simulink model "sampleModel1505"  (R2023a)
settings: Solver=VariableStepAuto  StartTime=0.0  StopTime=10.0  RelTol=1e-3
libraries: hdlsllib x11, simulink x2
settings Model: Creator=user1  LastModifiedBy=user1

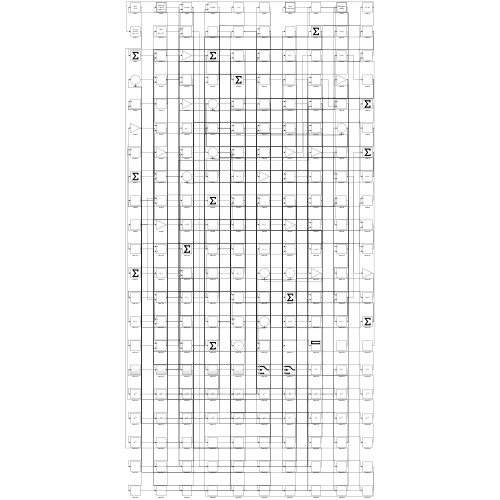
[thumbnail: Simulink's stored preview of the top-level diagram]
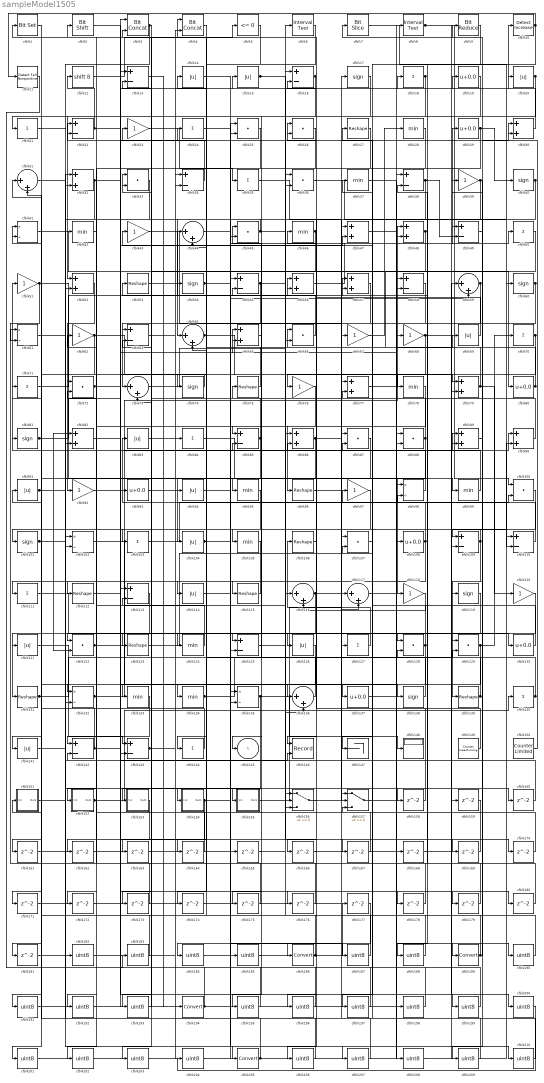
== system sampleModel1505 ==
  cfblk1 : simulink/Logic and Bit Operations/Bit Set  iBit=0
      settings: LibrarySourceBlock=|
      | hdlsllib/Logic and Bit
      | Operations/Bit Set
  cfblk10 : simulink/Logic and Bit Operations/Detect Increase  vinit=0.0  OutDataTypeStr=boolean
      settings: LibrarySourceBlock=|
      | hdlsllib/Logic and Bit
      | Operations/Detect
      | Increase
  cfblk{25..26,33,36,45,66,72,87..88,100,107,122,128..129} (14 alike) : DotProduct  OutDataTypeStr=Inherit: Inherit via internal rule
  cfblk{17,40,54,60,74,81,101,119,138} (9 alike) : Signum
  cfblk{41,61,98,102,132,135} (6 alike) : Product  Inputs=*/  RndMeth=Zero  SaturateOnIntegerOverflow=on
  cfblk{18,21,24,35,50,70..71,84,103,111,127,140,144} (13 alike) : Sum  Inputs=+
  cfblk{14..15,20,69,83,91,94,104,114,121,126,141} (12 alike) : Abs  SaturateOnIntegerOverflow=off
  cfblk{28,37,42,46,78,95,99,105,124,133..134} (11 alike) : MinMax
  cfblk{27,53,75,96,106,112,115,123,131,139} (10 alike) : Reshape
  cfblk{19,29,80,93,108,130,137} (7 alike) : Bias  Bias=0.0  SaturateOnIntegerOverflow=off
  cfblk{13,16,22,34,38,49,55,58,63,85,109..110,113,125,142..143} (16 alike) : Sum  Inputs=+-
  cfblk11 : hdlsllib/Logic and Bit Operations/Detect Fall Nonpositive  vinit=0  OutDataTypeStr=boolean
  cfblk{31,44,59,64,73,116..117,136} (8 alike) : Sum  Inputs=|++
  cfblk{23,39,43,51,62,67..68,76,92,97,118,120} (12 alike) : Gain
  cfblk12 : ArithShift  BitShiftNumber=8
  cfblk146 : Record  FileSettingsInternal="{\"entries\":[{\"content\":{\"excelSettings\":{\"content\":{},\"type\":\"Streamout.ExcelSettings\"}},\"type\":\"Streamout.FileSettingStorage\",\"uuid\":\"\"}],\"packageUris\":[\"http:\\/\\/schema.mathworks.com\\/mf0\\/streamout_blocks\\/R2020a\"],\"version\":\"1.0\"}"  Layout=[1 1]  SignalsInternal="{\"entries\":[{\"content\":{\"signals\":[{\"content\":{\"blockPath\":[],\"dimensions\":[1],\"domain\":\"\",\"lineColor\":\"#a2142f\",\"plots\":[1],\"port\":1,\"signalID\":1371,\"signalName\":\"XY Graph:1\"},\"type\":\"RecordBlkView.Signal\",\"uuid\":\"\"},{\"content\":{\"blockPath\":[],\"dimensions\":[1],\"domain\":\"\",\"lineColor\":\"#139fff\",\"plots\":[1],\"port\":2,\"signalID\":1374,\"signalName\":\"XY Graph:2\"},\"type\":\"RecordBlkView.Signal\",\"uuid\":\"\"}]},\"type\":\"RecordBlkView.InputSignals\",\"uuid\":\"\"}],\"packageUris\":[\"http:\\/\\/schema.mathworks.com\\/mf0\\/streamout_blocks\\/R2020a\"],\"version\":\"1.0\"}"  VisualizationBindings="{\"xyplotplugin\":{\"info\":[{\"series\":[{\"bindingParametersList\":[{\"parameter\":\"X-Axis\",\"signalID\":1371,\"signalName\":\"XY Graph:1\"},{\"parameter\":\"Y-Axis\",\"signalID\":1374,\"signalName\":\"XY Graph:2\"}],\"seriesID\":50908}],\"subplotID\":1}]}}"  CompatibilityTag=XY  st=-1
  cfblk147 : Terminator
  cfblk148 : Display
  cfblk149 : hdlsllib/Sources/Counter Free-Running  NumBits=16  tsamp=-1
  cfblk150 : hdlsllib/Sources/Counter Limited  uplimit=7  tsamp=-1
  cfblk151 : Subsystem
      settings: LibrarySourceBlock=|
      | hdlsllib/Ports &
      | Subsystems/Subsystem
  cfblk152 : Subsystem
      settings: LibrarySourceBlock=|
      | hdlsllib/Ports &
      | Subsystems/Subsystem
  cfblk153 : Subsystem
      settings: LibrarySourceBlock=|
      | hdlsllib/Ports &
      | Subsystems/Subsystem
  cfblk154 : Subsystem
      settings: LibrarySourceBlock=|
      | hdlsllib/Ports &
      | Subsystems/Subsystem
  cfblk155 : Subsystem
      settings: LibrarySourceBlock=|
      | hdlsllib/Ports &
      | Subsystems/Subsystem
  cfblk156 : Switch  SaturateOnIntegerOverflow=off  InputSameDT=off
  cfblk157 : Switch  SaturateOnIntegerOverflow=off  InputSameDT=off
  cfblk{158..181} (24 alike) : Delay  SampleTime=1
  cfblk{182..185,187..188,190..193,195..204,206..210} (25 alike) : DataTypeConversion  OutDataTypeStr=uint8  SaturateOnIntegerOverflow=off  RndMeth=Floor
  cfblk{186,189,194,205} (4 alike) : DataTypeConversion  SaturateOnIntegerOverflow=off  RndMeth=Floor
  cfblk2 : hdlsllib/Logic and Bit Operations/Bit Shift  mode=Shift Left Logical  N=0
  cfblk3 : hdlsllib/Logic and Bit Operations/Bit Concat  numInputs=2
  cfblk{30,32,47..48,52,56..57,65,77,79,82,86,89..90} (14 alike) : Sum
  cfblk4 : hdlsllib/Logic and Bit Operations/Bit Concat  numInputs=2
  cfblk5 : hdlsllib/Logic and Bit Operations/Compare To Zero  relop=<=  OutDataTypeStr=boolean
  cfblk6 : hdlsllib/Logic and Bit Operations/Interval Test  IntervalClosedRight=on  uplimit=0.5  IntervalClosedLeft=on  lowlimit=-0.5  OutDataTypeStr=boolean
  cfblk7 : hdlsllib/Logic and Bit Operations/Bit Slice  lidx=7  ridx=0
  cfblk8 : hdlsllib/Logic and Bit Operations/Interval Test  IntervalClosedRight=on  uplimit=0.5  IntervalClosedLeft=on  lowlimit=-0.5  OutDataTypeStr=boolean
  cfblk9 : hdlsllib/Logic and Bit Operations/Bit Reduce  mode=AND
  cfblk145 : Outport  VectorParamsAs1DForOutWhenUnconnected=off
  wires:
  cfblk52/1 -> cfblk92/1
  cfblk152/1(Out1) -> cfblk140/1, cfblk146/2, cfblk179/1
  cfblk67/1 -> cfblk28/1
  cfblk102/1 -> cfblk138/1
  cfblk103/1 -> cfblk97/1
  cfblk135/1 -> cfblk148/1, cfblk153/1(In1)
  cfblk91/1 -> cfblk99/1, cfblk122/2, cfblk82/1
  cfblk85/1 -> cfblk104/1, cfblk54/1
  cfblk140/1 -> cfblk75/1, cfblk129/2
  cfblk23/1 -> cfblk35/1
  cfblk48/1 -> cfblk65/1, cfblk128/1
  cfblk30/1 -> cfblk10/1
  cfblk19/1 -> cfblk52/1
  cfblk10/1 -> cfblk11/1, cfblk188/1
  cfblk137/1 -> cfblk50/1
  cfblk55/1 -> cfblk73/1, cfblk129/1
  cfblk90/1 -> cfblk33/1
  cfblk96/1 -> cfblk157/1
  cfblk149/1 -> cfblk53/1
  cfblk132/1 -> cfblk48/1, cfblk199/1
  cfblk70/1 -> cfblk76/1, cfblk79/1
  cfblk75/1 -> cfblk22/1
  cfblk150/1 -> cfblk7/1
  cfblk13/1 -> cfblk194/1
  cfblk38/1 -> cfblk64/1, cfblk49/2
  cfblk41/1 -> cfblk80/1
  cfblk93/1 -> cfblk18/1
  cfblk111/1 -> cfblk125/1
  cfblk53/1 -> cfblk127/1
  cfblk12/1 -> cfblk5/1
  cfblk26/1 -> cfblk144/1
  cfblk3/1 -> cfblk133/1, cfblk132/2
  cfblk110/1 -> cfblk46/1
  cfblk43/1 -> cfblk117/1
  cfblk31/1 -> cfblk205/1
  cfblk8/1 -> cfblk100/1, cfblk190/1
  cfblk127/1 -> cfblk106/1
  cfblk71/1 -> cfblk44/1
  cfblk81/1 -> cfblk65/2, cfblk160/1
  cfblk56/1 -> cfblk29/1
  cfblk73/1 -> cfblk6/1
  cfblk51/1 -> cfblk118/1, cfblk61/2
  cfblk123/1 -> cfblk17/1
  cfblk21/1 -> cfblk52/2
  cfblk64/1 -> cfblk117/2, cfblk79/2
  cfblk7/1 -> cfblk60/1
  cfblk40/1 -> cfblk63/1, cfblk156/3, cfblk195/1
  cfblk9/1 -> cfblk137/1
  cfblk46/1 -> cfblk73/2, cfblk103/1
  cfblk121/1 -> cfblk143/1
  cfblk80/1 -> cfblk4/1, cfblk66/1
  cfblk66/1 -> cfblk56/1
  cfblk130/1 -> cfblk43/1
  cfblk72/1 -> cfblk134/1, cfblk126/1
  cfblk74/1 -> cfblk72/1
  cfblk129/1 -> cfblk147/1, cfblk70/1, cfblk175/1
  cfblk35/1 -> cfblk67/1
  cfblk139/1 -> cfblk9/1, cfblk38/2
  cfblk15/1 -> cfblk169/1, cfblk170/1
  cfblk88/1 -> cfblk125/2, cfblk63/2
  cfblk45/1 -> cfblk42/1, cfblk136/2
  cfblk124/1 -> cfblk62/1
  cfblk37/1 -> cfblk189/1
  cfblk120/1 -> cfblk122/1
  cfblk4/1 -> cfblk74/1
  cfblk89/1 -> cfblk109/1
  cfblk101/1 -> cfblk201/1, cfblk207/1
  cfblk116/1 -> cfblk131/1, cfblk89/1, cfblk163/1
  cfblk112/1 -> cfblk47/2
  cfblk106/1 -> cfblk56/2
  cfblk29/1 -> cfblk95/1, cfblk40/1
  cfblk104/1 -> cfblk30/2, cfblk176/1
  cfblk24/1 -> cfblk130/1
  cfblk76/1 -> cfblk96/1
  cfblk39/1 -> cfblk108/1, cfblk136/1, cfblk119/1
  cfblk16/1 -> cfblk102/2, cfblk32/2
  cfblk94/1 -> cfblk90/1
  cfblk34/1 -> cfblk3/2
  cfblk63/1 -> cfblk57/1
  cfblk61/1 -> cfblk154/1(In1)
  cfblk6/1 -> cfblk44/2
  cfblk42/1 -> cfblk22/2
  cfblk69/1 -> cfblk26/1
  cfblk155/1(Out1) -> cfblk49/1
  cfblk22/1 -> cfblk78/1, cfblk12/1
  cfblk156/1 -> cfblk19/1
  cfblk118/1 -> cfblk116/2
  cfblk2/1 -> cfblk143/2
  cfblk115/1 -> cfblk114/1
  cfblk138/1 -> cfblk45/1
  cfblk143/1 -> cfblk34/2, cfblk20/1
  cfblk84/1 -> cfblk156/1
  cfblk99/1 -> cfblk58/1
  cfblk1/1 -> cfblk111/1
  cfblk60/1 -> cfblk88/2, cfblk124/1
  cfblk87/1 -> cfblk186/1
  cfblk57/1 -> cfblk157/2
  cfblk122/1 -> cfblk58/2, cfblk167/1
  cfblk32/1 -> cfblk26/2, cfblk15/1, cfblk82/2
  cfblk134/1 -> cfblk8/1, cfblk100/2, cfblk180/1
  cfblk54/1 -> cfblk59/2, cfblk66/2, cfblk178/1
  cfblk27/1 -> cfblk115/1
  cfblk128/1 -> cfblk85/2, cfblk196/1
  cfblk65/1 -> cfblk145/1
  cfblk68/1 -> cfblk146/1, cfblk110/2
  cfblk36/1 -> cfblk110/1
  cfblk133/1 -> cfblk142/1
  cfblk98/1 -> cfblk51/1
  cfblk131/1 -> cfblk81/1, cfblk59/1
  cfblk62/1 -> cfblk135/1, cfblk121/1
  cfblk154/1(Out1) -> cfblk173/1, cfblk210/1
  cfblk144/1 -> cfblk71/1
  cfblk78/1 -> cfblk112/1
  cfblk83/1 -> cfblk55/2
  cfblk59/1 -> cfblk105/1, cfblk135/2
  cfblk141/1 -> cfblk155/1(In1)
  cfblk92/1 -> cfblk86/2
  cfblk142/1 -> cfblk41/1, cfblk30/1
  cfblk114/1 -> cfblk48/2
  cfblk136/1 -> cfblk64/2
  cfblk108/1 -> cfblk83/1, cfblk27/1, cfblk132/1, cfblk93/1
  cfblk117/1 -> cfblk69/1
  cfblk79/1 -> cfblk24/1, cfblk120/1
  cfblk47/1 -> cfblk98/1
  cfblk86/1 -> cfblk141/1, cfblk16/2, cfblk89/2
  cfblk82/1 -> cfblk68/1
  cfblk109/1 -> cfblk139/1, cfblk101/1
  cfblk95/1 -> cfblk152/1(In1)
  cfblk20/1 -> cfblk85/1, cfblk45/2
  cfblk50/1 -> cfblk123/1
  cfblk18/1 -> cfblk36/2, cfblk21/1
  cfblk125/1 -> cfblk158/1
  cfblk158/1 -> cfblk1/1
  cfblk159/1 -> cfblk157/3
  cfblk160/1 -> cfblk102/1
  cfblk105/1 -> cfblk161/1
  cfblk161/1 -> cfblk116/1
  cfblk153/1(Out1) -> cfblk162/1
  cfblk162/1 -> cfblk86/1
  cfblk17/1 -> cfblk164/1
  cfblk164/1 -> cfblk142/2
  cfblk44/1 -> cfblk165/1
  cfblk165/1 -> cfblk16/1
  cfblk58/1 -> cfblk166/1
  cfblk166/1 -> cfblk109/2
  cfblk167/1 -> cfblk156/2
  cfblk169/1 -> cfblk34/1
  cfblk170/1 -> cfblk98/2
  cfblk97/1 -> cfblk171/1
  cfblk171/1 -> cfblk47/1
  cfblk33/1 -> cfblk172/1
  cfblk172/1 -> cfblk4/2
  cfblk173/1 -> cfblk61/1
  cfblk5/1 -> cfblk174/1
  cfblk174/1 -> cfblk57/2
  cfblk175/1 -> cfblk55/1
  cfblk176/1 -> cfblk72/2
  cfblk178/1 -> cfblk2/1
  cfblk179/1 -> cfblk128/2
  cfblk180/1 -> cfblk41/2
  cfblk126/1 -> cfblk181/1
  cfblk181/1 -> cfblk3/1
  cfblk151/1(Out1) -> cfblk182/1
  cfblk182/1 -> cfblk94/1
  cfblk11/1 -> cfblk183/1
  cfblk183/1 -> cfblk151/1(In1)
  cfblk177/1 -> cfblk184/1
  cfblk14/1 -> cfblk185/1
  cfblk185/1 -> cfblk177/1
  cfblk186/1 -> cfblk14/1, cfblk36/1
  cfblk184/1 -> cfblk187/1
  cfblk187/1 -> cfblk87/1
  cfblk188/1 -> cfblk87/2
  cfblk189/1 -> cfblk39/1, cfblk91/1
  cfblk190/1 -> cfblk37/1
  cfblk113/1 -> cfblk191/1
  cfblk191/1 -> cfblk88/1
  cfblk100/1 -> cfblk192/1
  cfblk192/1 -> cfblk113/1
  cfblk163/1 -> cfblk193/1
  cfblk193/1 -> cfblk113/2
  cfblk194/1 -> cfblk33/2, cfblk38/1
  cfblk195/1 -> cfblk13/1
  cfblk196/1 -> cfblk13/2
  cfblk107/1 -> cfblk197/1
  cfblk197/1 -> cfblk23/1
  cfblk157/1 -> cfblk198/1
  cfblk198/1 -> cfblk107/1
  cfblk199/1 -> cfblk107/2
  cfblk168/1 -> cfblk200/1
  cfblk201/1 -> cfblk168/1
  cfblk25/1 -> cfblk202/1
  cfblk202/1 -> cfblk84/1
  cfblk28/1 -> cfblk203/1
  cfblk203/1 -> cfblk25/1
  cfblk200/1 -> cfblk204/1
  cfblk204/1 -> cfblk25/2
  cfblk205/1 -> cfblk90/2, cfblk32/1
  cfblk119/1 -> cfblk206/1
  cfblk206/1 -> cfblk31/1
  cfblk207/1 -> cfblk31/2
  cfblk77/1 -> cfblk208/1
  cfblk208/1 -> cfblk159/1
  cfblk49/1 -> cfblk209/1
  cfblk209/1 -> cfblk77/1
  cfblk210/1 -> cfblk77/2

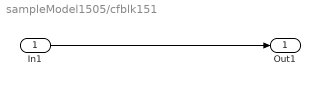
== system sampleModel1505/cfblk151 ==
  In1 : Inport
  Out1 : Outport
  wires:
  In1/1 -> Out1/1

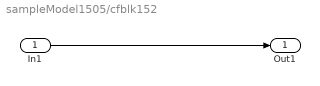
== system sampleModel1505/cfblk152 ==
  In1 : Inport
  Out1 : Outport
  wires:
  In1/1 -> Out1/1

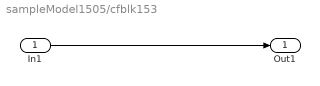
== system sampleModel1505/cfblk153 ==
  In1 : Inport
  Out1 : Outport
  wires:
  In1/1 -> Out1/1

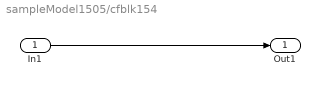
== system sampleModel1505/cfblk154 ==
  In1 : Inport
  Out1 : Outport
  wires:
  In1/1 -> Out1/1

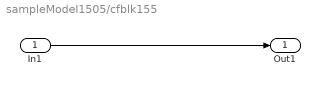
== system sampleModel1505/cfblk155 ==
  In1 : Inport
  Out1 : Outport
  wires:
  In1/1 -> Out1/1
